simulink library "parking_algorithm_atomic_sub_chart_library"  (R2013b)
settings: Solver=ode45  StartTime=0.0  StopTime=10.0  RelTol=1e-3
settings Model: Creator=mbiesiad  LastModifiedBy=grouleau

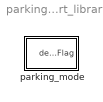
== system parking_algorithm_atomic_sub_chart_library ==
  parking_mode : Stateflow chart  TreatAsAtomicUnit=on

== stateflow chart parking_algorithm_atomic_sub_chart_library/parking_mode ==
  state parking_mode
    entry: debugFlag = uint16(800);
  data: debugFlag output uint16 size=1
